simulink model "mCSControls_DG"  (R2012b)
settings: Solver=FixedStepDiscrete  StartTime=0.0  StopTime=10.0  RelTol=1e-3
values from neighbouring files (symbols this model uses):
  CDF2FThreshold = 45    [ControlCal_DG.m]
  CDF2TempThreshold = 20    [ControlCal_DG.m]
  delay = 5    [ControlCal_DG.m]
  DFThresh = 33    [ControlCal_DG.m]
  H = [90 90 90 90]    [ControlCal_DG.m]
  HeatTempThresh1 = 40    [ControlCal_DG.m]
  HeatTempThresh2 = 30    [ControlCal_DG.m]
  HeatTempThresh3 = 20    [ControlCal_DG.m]
  HStabilizationTime = 2*60    (= 120)    [ControlCal_DG.m]
  I_FAN = -1    [ControlCal_DG.m]
  I_VALVE = -1    [ControlCal_DG.m]
  initialSet = [1 1 1]    [ControlCal_DG.m]
  PBFTempThreshold = 30    [ControlCal_DG.m]
  PowerModeSwitchDelay = 30    [ControlCal_DG.m]
  SVocThresh = 550    [ControlCal_DG.m]
  T = [0 4 7 10]    [ControlCal_DG.m]
  Ts = 0.5    [ControlCal_DG.m]
  TSTempSetPoint = -2    [ControlCal_DG.m]
  TV1FThresh = 45    [ControlCal_DG.m]
  TV2FThresh = 60    [ControlCal_DG.m]
  VbatThresh = 22    [ControlCal_DG.m]
  VocDecRate = 0.5    [ControlCal_DG.m]
  VocIncrement = 5    [ControlCal_DG.m]
libraries: c2833xlib x29, simulink x23, c280xlib x11, idelinklib_tgtpref x1
(part 3 of 4)

== system mCSControls_DG/Inputs/DriveParams/DriveParamReceive/Rx/OPFreqRx ==
  SCIBRx : Inport
  Enable : EnablePort
  CRC-16L : Terminator
  CRC-16U : Terminator
  Data Type Conversion : DataTypeConversion  OutDataTypeStr=double
  Data Type Conversion1 : DataTypeConversion  OutDataTypeStr=uint16
  DataQuantity : Terminator
  Demux : Demux  Outputs=15
  FunctionCount : Terminator
  Gain : Gain  Gain=256  OutDataTypeStr=uint16
  Gain1 : Gain  Gain=0.01
  Loopback{1..8} (8 alike) : Terminator
  SlaveAddress : Terminator
  Sum : Sum  Inputs=|++
  D : Outport
  wires:
  Data Type Conversion1/1 -> Gain/1
  SCIBRx/1 -> Demux/1
  Gain/1 -> Sum/1
  Demux/1 -> Loopback1/1
  Demux/2 -> Loopback2/1
  Demux/3 -> Loopback3/1
  Demux/4 -> Loopback4/1
  Demux/5 -> Loopback5/1
  Demux/6 -> Loopback6/1
  Demux/7 -> Loopback7/1
  Demux/8 -> Loopback8/1
  Demux/9 -> SlaveAddress/1
  Demux/10 -> FunctionCount/1
  Demux/11 -> DataQuantity/1
  Demux/15 -> CRC-16L/1
  Demux/14 -> CRC-16U/1
  Demux/12 -> Data Type Conversion1/1
  Demux/13 -> Sum/2
  Sum/1 -> Data Type Conversion/1  "PFreq"
  Data Type Conversion/1 -> Gain1/1
  Gain1/1 -> D/1

== stateflow chart mCSControls_DG/Outputs/EEPROM/OneSecTimer ==
  state NoTrigger
    en,du: Enable=0;
  state DataChanged
    en,du: Enable=0;
  state Triggered
    en,du: Enable=1;
  (default) -> NoTrigger
  Triggered -> NoTrigger [order 2]
  NoTrigger -> DataChanged : [Input>0]
  Triggered -> DataChanged [order 1] : [Input>0]
  DataChanged -> Triggered : [Reading==0]
  data: Input input uint16; Enable output double [0..1]; Reading input double

== system mCSControls_DG/Inputs/DriveParams/DriveParamReceive/Rx/OPPowerRx ==
  SCIBRx : Inport
  Enable : EnablePort
  CRC-16L : Terminator
  CRC-16U : Terminator
  Data Type Conversion : DataTypeConversion  OutDataTypeStr=double
  Data Type Conversion1 : DataTypeConversion  OutDataTypeStr=uint16
  DataQuantity : Terminator
  Demux : Demux  Outputs=15
  FunctionCount : Terminator
  Gain : Gain  Gain=256  OutDataTypeStr=uint16
  Gain1 : Gain  Gain=0.01
  Loopback{1..8} (8 alike) : Terminator
  SlaveAddress : Terminator
  Sum : Sum  Inputs=|++
  D : Outport
  wires:
  Demux/13 -> Sum/2
  Demux/12 -> Data Type Conversion1/1
  Demux/14 -> CRC-16U/1
  Demux/15 -> CRC-16L/1
  Demux/11 -> DataQuantity/1
  Demux/10 -> FunctionCount/1
  Demux/9 -> SlaveAddress/1
  Demux/8 -> Loopback8/1
  Demux/7 -> Loopback7/1
  Demux/6 -> Loopback6/1
  Demux/5 -> Loopback5/1
  Demux/4 -> Loopback4/1
  Demux/3 -> Loopback3/1
  Demux/2 -> Loopback2/1
  Demux/1 -> Loopback1/1
  Gain/1 -> Sum/1
  SCIBRx/1 -> Demux/1
  Data Type Conversion1/1 -> Gain/1
  Data Type Conversion/1 -> Gain1/1
  Sum/1 -> Data Type Conversion/1  "PFreq"
  Gain1/1 -> D/1

== system mCSControls_DG/Inputs/DriveParams/DriveParamReceive/TxAndDE_RE_Zero/DE_RE_Zero ==
  Trigger : TriggerPort  TriggerType=falling  PortDimensions=1
  DE : Constant  SampleTime=-1
  Digital Output : c2833xlib/Digital Output  GPIO_Number=GPIO0~GPIO7  GPIO_Bit0=off  GPIO_BIT0_Toggle=off  GPIO_Bit1=off  GPIO_BIT1_Toggle=off  GPIO_Bit2=off  GPIO_BIT2_Toggle=off  GPIO_Bit3=off  GPIO_BIT3_Toggle=off  GPIO_Bit4=off  GPIO_BIT4_Toggle=off  GPIO_Bit5=off  GPIO_BIT5_Toggle=off  GPIO_Bit6=off  GPIO_BIT6_Toggle=off  GPIO_Bit7=on  GPIO_BIT7_Toggle=off
  Digital Output1 : c2833xlib/Digital Output  GPIO_Number=GPIO48~GPIO55  GPIO_Bit0=off  GPIO_BIT0_Toggle=off  GPIO_Bit1=on  GPIO_BIT1_Toggle=off  GPIO_Bit2=off  GPIO_BIT2_Toggle=off  GPIO_Bit3=off  GPIO_BIT3_Toggle=off  GPIO_Bit4=off  GPIO_BIT4_Toggle=off  GPIO_Bit5=off  GPIO_BIT5_Toggle=off  GPIO_Bit6=off  GPIO_BIT6_Toggle=off  GPIO_Bit7=off  GPIO_BIT7_Toggle=off
  RE : Constant  Value=0  SampleTime=-1
  wires:
  DE/1 -> Digital Output/1
  RE/1 -> Digital Output1/1

== system mCSControls_DG/Inputs/DriveParams/DriveParamReceive/TxAndDE_RE_Zero/FAULTSTx ==
  CRC-16 : Constant  Value=13268 % D433H
  Data Type Conversion : DataTypeConversion  OutDataTypeStr=uint16  RndMeth=Simplest
  Mux : Mux
  Quantity : Constant  Value=256 % 0001H
  SlaveAddressFunctionCode : Constant  Value=770 % 0203H
  StartingNumber : Constant  Value=8448 % 0021H
  SCIBTx : Outport
  wires:
  Quantity/1 -> Mux/3
  StartingNumber/1 -> Mux/2
  SlaveAddressFunctionCode/1 -> Mux/1
  CRC-16/1 -> Mux/4
  Data Type Conversion/1 -> SCIBTx/1
  Mux/1 -> Data Type Conversion/1

== system mCSControls_DG/Inputs/DriveParams/DriveParamReceive/TxAndDE_RE_Zero/OPCurrTx ==
  CRC-16 : Constant  Value=62053 % 65F2H
  Data Type Conversion : DataTypeConversion  OutDataTypeStr=uint16  RndMeth=Simplest
  Mux : Mux
  Quantity : Constant  Value=256 % 0001H
  SlaveAddressFunctionCode : Constant  Value=770 % 0203H
  StartingNumber : Constant  Value=9728 % 0026H
  SCIBTx : Outport
  wires:
  Quantity/1 -> Mux/3
  StartingNumber/1 -> Mux/2
  SlaveAddressFunctionCode/1 -> Mux/1
  CRC-16/1 -> Mux/4
  Data Type Conversion/1 -> SCIBTx/1
  Mux/1 -> Data Type Conversion/1

== system mCSControls_DG/Inputs/DriveParams/DriveParamReceive/TxAndDE_RE_Zero/OPFreqTx ==
  CRC-16 : Constant  Value=12996 % C432H
  Data Type Conversion : DataTypeConversion  OutDataTypeStr=uint16  RndMeth=Simplest
  Mux : Mux
  Quantity : Constant  Value=256 % 0001H
  SlaveAddressFunctionCode : Constant  Value=770 % 0203H
  StartingNumber : Constant  Value=9216 % 0024H
  SCIBTx : Outport
  wires:
  Mux/1 -> Data Type Conversion/1
  Data Type Conversion/1 -> SCIBTx/1
  CRC-16/1 -> Mux/4
  SlaveAddressFunctionCode/1 -> Mux/1
  StartingNumber/1 -> Mux/2
  Quantity/1 -> Mux/3

== system mCSControls_DG/Inputs/DriveParams/DriveParamReceive/TxAndDE_RE_Zero/OPPowerTx ==
  CRC-16 : Constant  Value=12852 % 3432H
  Data Type Conversion : DataTypeConversion  OutDataTypeStr=uint16  RndMeth=Simplest
  Mux : Mux
  Quantity : Constant  Value=256 % 0001H
  SlaveAddressFunctionCode : Constant  Value=770 % 0203H
  StartingNumber : Constant  Value=9984 % 0027H
  SCIBTx : Outport
  wires:
  Mux/1 -> Data Type Conversion/1
  Data Type Conversion/1 -> SCIBTx/1
  CRC-16/1 -> Mux/4
  SlaveAddressFunctionCode/1 -> Mux/1
  StartingNumber/1 -> Mux/2
  Quantity/1 -> Mux/3

== system mCSControls_DG/Inputs/DriveParams/DriveParamReceive/TxAndDE_RE_Zero/SCI B Tx ==
  In1 : Inport
  Trigger : TriggerPort  PortDimensions=1
  SCI B Transmit : c280xlib/SCI Transmit  sciModule=B  dataHead=''  dataTail=''  postInterrupt=off  numFifo=1
  wires:
  In1/1 -> SCI B Transmit/1
